simulink model "full"  (R2022a)
settings: Solver=VariableStepAuto  StartTime=0.0  StopTime=0.1  RelTol=1e-3
libraries: spsSeriesRLCBranchLib x7, spsVoltageMeasurementLib x6, spsCurrentMeasurementLib x5, spsIGBTDiodeLib x5, simulink x2, spsDiodeLib x1, spsPVArrayLib x1, spspowerguiLib x1
settings Model: Creator=nikke  LastModifiedBy=nikke

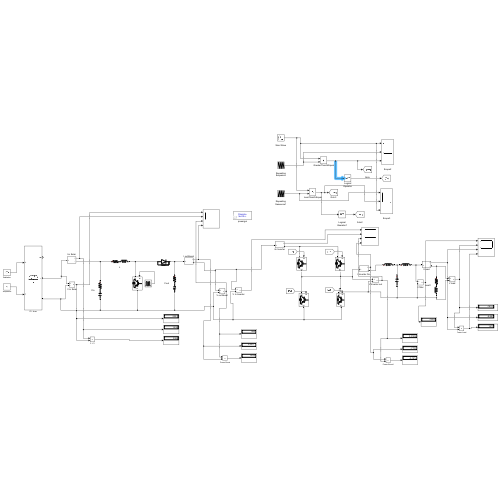
[thumbnail: Simulink's stored preview of the top-level diagram]
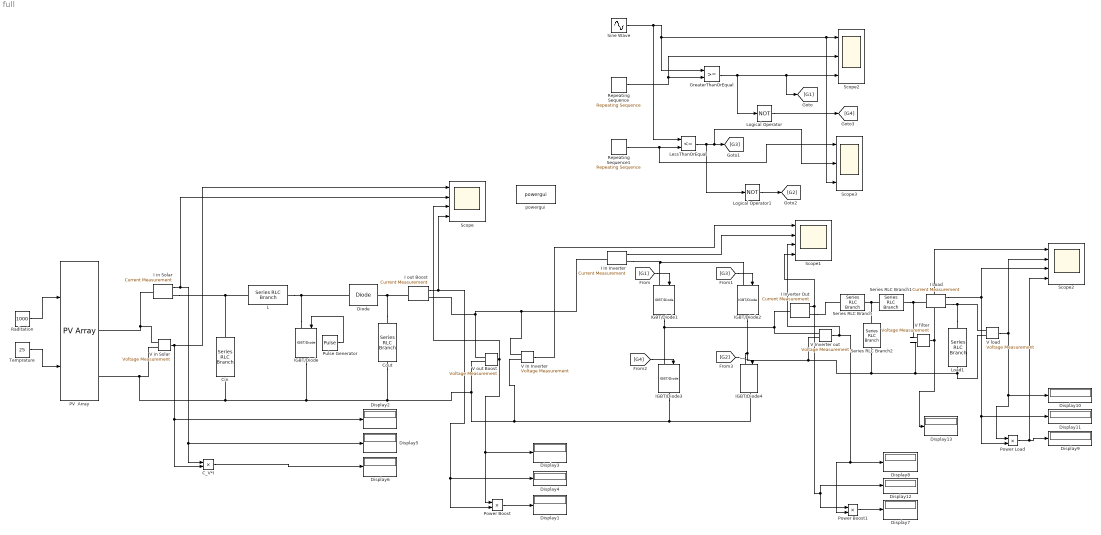
== system full ==
  " Logical Operator1" : Logic  Operator=NOT  AllPortsSameDT=off  OutDataTypeStr=boolean
  " Repeating Sequence" : simulink/Sources/Repeating Sequence  rep_seq_t=[0 1/2 1]*(1/1500)  rep_seq_y=[0 1 0]
  " Repeating Sequence1" : simulink/Sources/Repeating Sequence  rep_seq_t=[0 1/2 1]*(1/1500)  rep_seq_y=[0 -1 0]
  " Scope3" : Scope  NumInputPorts=3
  " Sine Wave" : Sin  Amplitude=0.98  Frequency=2*pi*50  SampleTime=0
  " Scope2" : Scope  NumInputPorts=3
  " GreaterThanOrEqual" : RelationalOperator  OutDataTypeStr=boolean  RndMeth=Simplest  InputSameDT=off
  " LessThanOrEqual" : RelationalOperator  Operator=<=  OutDataTypeStr=boolean  RndMeth=Simplest  InputSameDT=off
  " Logical Operator" : Logic  Operator=NOT  AllPortsSameDT=off  OutDataTypeStr=boolean
  " Power Boost" : Product
  " Power Boost1" : Product
  C_V*I : Product
  Cin : spsSeriesRLCBranchLib/Series RLC Branch  LConnTagsString=__new0  RConnTagsString=__new0  BranchType=RC  Resistance=1e-4  Inductance=1e-3  SetiL0=off  InitialCurrent=0  Capacitance=100e-6  Setx0=off  InitialVoltage=0  Measurements=None
  Cout : spsSeriesRLCBranchLib/Series RLC Branch  LConnTagsString=__new0  RConnTagsString=__new0  BranchType=RC  Resistance=0.0001  Inductance=1e-3  SetiL0=off  InitialCurrent=0  Capacitance=100e-6  Setx0=off  InitialVoltage=0  Measurements=None
  Diode : spsDiodeLib/Diode  Ron=0.001  Lon=0  Vf=0.8  IC=0  UseSnubber=off  Rs=500  Cs=250e-9  Measurements=off
  Display{1..13} (13 alike) : Display
  "I In Inverter " : spsCurrentMeasurementLib/Current Measurement  PhasorSimulation=off  OutputType=Complex  PSBequivalent=0
  I Inverter Out : spsCurrentMeasurementLib/Current Measurement  PhasorSimulation=off  OutputType=Complex  PSBequivalent=0
  I Load : spsCurrentMeasurementLib/Current Measurement  PhasorSimulation=off  OutputType=Complex  PSBequivalent=0
  I in Solar : spsCurrentMeasurementLib/Current Measurement  PhasorSimulation=off  OutputType=Complex  PSBequivalent=0
  I out Boost : spsCurrentMeasurementLib/Current Measurement  PhasorSimulation=off  OutputType=Complex  PSBequivalent=0
  IGBT/Diode{,1..4} (5 alike) : spsIGBTDiodeLib/IGBT//Diode  Ron=1e-3  Rs=1e5  Cs=inf  Measurements=off
  L : spsSeriesRLCBranchLib/Series RLC Branch  LConnTagsString=__new0  RConnTagsString=__new0  BranchType=RL  Resistance=0.1  Inductance=2e-3  SetiL0=off  InitialCurrent=0  Capacitance=100e-6  Setx0=off  InitialVoltage=0  Measurements=None
  Load1 : spsSeriesRLCBranchLib/Series RLC Branch  LConnTagsString=__new0  RConnTagsString=__new0  BranchType=RL  Resistance=27  Inductance=200e-3  SetiL0=off  InitialCurrent=0  Capacitance=100e-6  Setx0=off  InitialVoltage=0  Measurements=None
  PV  Array : spsPVArrayLib/PV Array  Npar=2  Nser=12  PlotType=array @ 1000 W/m2 & specified temperatures  S_vec="[ 1000  500  100 ]"  Temp_C_vec="[ 45 25  ]"  ModuleName=Tata Power Solar Systems TP140SBZ  PlotWhenSelected=off  Pm=139.6944  Ncell=36  Voc=22.25  Isc=8.66  Vm=17.44  Im=8.01  beta_Voc_pc=-0.33  alpha_Isc_pc=0.063799  beta_Voc=-0.073425  alpha_Isc=0.005525  IL=8.6872  I0=9.8965e-11  nI=0.95579  Rsh=88.7762  Rs=0.27837  RobustModel=off  RobustCellTemperature=313.3991  BAL=on  Tc=1e-6  Tfilter=5e-5
  Power Load : Product
  Pulse Generator : DiscretePulseGenerator  PulseType=Time based  Period=1/1000  PulseWidth=50
  Raditation : Constant  Value=1000
  Scope : Scope  NumInputPorts=4
  Scope1 : Scope  NumInputPorts=4
  Scope2 : Scope  NumInputPorts=4
  Series RLC Branch : spsSeriesRLCBranchLib/Series RLC Branch  LConnTagsString=__new0  RConnTagsString=__new0  BranchType=L  Resistance=1  Inductance=200e-3  SetiL0=off  InitialCurrent=0  Capacitance=1e-6  Setx0=off  InitialVoltage=0  Measurements=None
  Series RLC Branch1 : spsSeriesRLCBranchLib/Series RLC Branch  LConnTagsString=__new0  RConnTagsString=__new0  BranchType=L  Resistance=1  Inductance=200e-3  SetiL0=off  InitialCurrent=0  Capacitance=1e-6  Setx0=off  InitialVoltage=0  Measurements=None
  Series RLC Branch2 : spsSeriesRLCBranchLib/Series RLC Branch  LConnTagsString=__new0  RConnTagsString=__new0  BranchType=C  Resistance=1  Inductance=1e-3  SetiL0=off  InitialCurrent=0  Capacitance=1e-6  Setx0=off  InitialVoltage=0  Measurements=None
  Temprature : Constant  Value=25
  "V In Inverter " : spsVoltageMeasurementLib/Voltage Measurement  PhasorSimulation=off  OutputType=Complex  PSBequivalent=0
  V Inverter out : spsVoltageMeasurementLib/Voltage Measurement  PhasorSimulation=off  OutputType=Complex  PSBequivalent=0
  V filter : spsVoltageMeasurementLib/Voltage Measurement  PhasorSimulation=off  OutputType=Complex  PSBequivalent=0
  "V in Solar " : spsVoltageMeasurementLib/Voltage Measurement  PhasorSimulation=off  OutputType=Complex  PSBequivalent=0
  "V load " : spsVoltageMeasurementLib/Voltage Measurement  PhasorSimulation=off  OutputType=Complex  PSBequivalent=0
  "V out Boost " : spsVoltageMeasurementLib/Voltage Measurement  PhasorSimulation=off  OutputType=Complex  PSBequivalent=0
  powergui : spspowerguiLib/powergui  Priority=1  SimulationMode=Discrete  SampleTime=50e-6  frequency=50  Iterations=50  frequencyindice=0  Pbase=100e6  ErrMax=1e-4  UnitsV=kV  UnitsW=MW  buscounter=0  FunctionMessages=off  echomessages=off  EnableUseOfTLC=off  CurrentSourceSwitches=off  DisableSnubberDevices=off  DisableRonSwitches=off  DisableVfSwitches=off  DisplayEquations=off  AutomaticDiscreteSolvers=off  SolverType=Tustin/Backward Euler (TBE)  Interpol=off  ExternalGateDelay=off  methode=off  Ts=100  x0status=blocks  SPID=on  SwTol=0  HookPort=off  NonlinearTolerance=1e-4  nMaxIteration=100  ContinueOnMaxIteration=off  RestoreLinks=warning  ResistiveCurrentMeasurement=off  Frange=[0:2:500]  Ylog=off  Xlog=on  ShowGrid=off  save=off  variable=ZData  structure=0  ZoomFFT=off  StartTime=0.0  cycles=1  DisplayStyle=1  fundamental=60  FreqAxis=off  MaxFrequency=1000  frequencyindicesteady=1  RmsSteady=1  display=off
  wires:
  C_V*I/1 -> Display6/1
  Pulse Generator/1 -> IGBT/Diode/1
  "V out Boost "/1 -> Scope/3, Display3/1, " Power Boost"/1
  " Power Boost"/1 -> Display1/1
  I in Solar/1 -> Display5/1, C_V*I/1, Scope/2
  "V in Solar "/1 -> C_V*I/2, Display2/1, Scope/1
  Raditation/1 -> PV  Array/1
  I out Boost/1 -> Display4/1, " Power Boost"/2, Scope/4
  Temprature/1 -> PV  Array/2
  " Logical Operator1"/1 -> [G2]
  " LessThanOrEqual"/1 -> " Logical Operator1"/1, " Scope3"/2, [G3]
  " GreaterThanOrEqual"/1 -> [G1], " Scope2"/3, " Logical Operator"/1
  " Logical Operator"/1 -> [G4]
  Power Load/1 -> Scope2/4, Display9/1
  [G1] -> IGBT/Diode1/1
  [G4] -> IGBT/Diode3/1
  " Sine Wave"/1 -> " LessThanOrEqual"/1, " GreaterThanOrEqual"/1, " Scope3"/3, " Scope2"/1
  "V load "/1 -> Scope2/2, Display10/1, Power Load/1
  [G3] -> IGBT/Diode2/1
  [G2] -> IGBT/Diode4/1
  I Load/1 -> Scope2/3, Display11/1, Power Load/2
  " Repeating Sequence1"/1 -> " Scope3"/1, " LessThanOrEqual"/2
  " Repeating Sequence"/1 -> " Scope2"/2, " GreaterThanOrEqual"/2
  I Inverter Out/1 -> Scope1/4, Display12/1, " Power Boost1"/1
  " Power Boost1"/1 -> Display7/1
  V Inverter out/1 -> Scope1/3, " Power Boost1"/2, Display8/1
  "V In Inverter "/1 -> Scope1/1
  "I In Inverter "/1 -> Scope1/2
  V filter/1 -> Display13/1, Scope2/1
  connections:
  I in Solar/RConn1 -- Cin/LConn1 -- L/LConn1
  Cout/LConn1 -- Diode/RConn1 -- I out Boost/LConn1
  "V in Solar "/LConn1 -- I in Solar/LConn1 -- PV  Array/RConn1
  IGBT/Diode/LConn1 -- L/RConn1 -- Diode/LConn1
  "V out Boost "/LConn1 -- I out Boost/RConn1 -- "V In Inverter "/LConn1 -- "I In Inverter "/LConn1
  Series RLC Branch/RConn1 -- Series RLC Branch1/LConn1 -- Series RLC Branch2/LConn1
  IGBT/Diode4/LConn1 -- V Inverter out/LConn2 -- V filter/LConn2 -- Load1/RConn1 -- "V load "/LConn2 -- Series RLC Branch2/RConn1 -- IGBT/Diode2/RConn1
  Load1/LConn1 -- "V load "/LConn1 -- I Load/RConn1
  "V out Boost "/LConn2 -- Cout/RConn1 -- "V in Solar "/LConn2 -- PV  Array/RConn2 -- Cin/RConn1 -- IGBT/Diode/RConn1 -- "V In Inverter "/LConn2 -- IGBT/Diode4/RConn1 -- IGBT/Diode3/RConn1
  IGBT/Diode1/RConn1 -- I Inverter Out/LConn1 -- V Inverter out/LConn1 -- IGBT/Diode3/LConn1
  "I In Inverter "/RConn1 -- IGBT/Diode2/LConn1 -- IGBT/Diode1/LConn1
  Series RLC Branch1/RConn1 -- V filter/LConn1 -- I Load/LConn1
  I Inverter Out/RConn1 -- Series RLC Branch/LConn1
